simulink model "Performance_QP_Simulink"  (R2021a)
settings: Solver=ode45  StartTime=0.0  StopTime=20  FixedStep=Control_timestep  RelTol=1e-3  AbsTol=1e-6
undefined symbols (not defined in the file): Matlab_version, NXMotion, NXMotion_controltimestep, NXMotion_model, NXMotion_model_n, NXMotion_n, NXMotion_solution, NXMotion_solution_n, Plant_inputs_num, Plant_outputs_num
libraries: simulink x1
(part 2 of 3)

== matlab function Performance_QP_Simulink/MATLAB Function5 ==
  data: A input; B input; Theta0 input; XB input; P0 input; dh input; g output; q input; J input
function g = Performance_Gradient(A, B, Theta0, XB, P0, dh, q, J)
% 当前优化指标：
%   1) 世界坐标系 z 方向的 Directional Force Manipulability
%   2) 世界坐标系 x-y 平面的 Directional Velocity Transmission
%   3) 世界坐标系 rx-ry 平面的 Directional Rotational Stiffness


    %% -------------------------------------------------
    % 0. 固定输出尺寸与输入整理
    % --------------------------------------------------
    g = zeros(13,1);

    mu_const = 5;

    q      = reshape(q,      13, 1);
    J      = reshape(J,       6, 13);
    A      = reshape(A,       6, 3);
    B      = reshape(B,       6, 3);
    XB     = reshape(XB,      3, 1);
    P0     = reshape(P0,      3, 1);
    dh     = reshape(dh,      7, 4);
    Theta0 = reshape(Theta0,  7, 1);

    theta7_fixed = 0.0;

    q(13)   = theta7_fixed;
    J(:,13) = 0.0;

    %% -------------------------------------------------
    % 1. 调参量
    % --------------------------------------------------
    dt = 1.0e-3;

    % z 方向 Directional Force Manipulability 权重
    w_m = 1;

    % rx-ry 方向 Rotational Stiffness 权重
    w_s = 0;

    % x-y 方向 Velocity Transmission 权重
    w_v = 0;

    % 离散加速度层缩放：
    %   q_{k+1} ≈ q_k + qdot_k*dt + 0.5*qddot_k*dt^2
    mu = mu_const * 0.5 * dt * dt;

    %% -------------------------------------------------
    % 2. 构造性能指标矩阵
    % --------------------------------------------------
    [S_tau, Kq_inv, S_qdot] = build_metric_mats_perf();

    %% -------------------------------------------------
    % 3. 当前构型下的 Jacobian 单位转换
    % --------------------------------------------------
    Jv_now = convert_Jv_force_velocity_units(J);
    Jk_now = convert_J_stiffness_units(J);

    %% -------------------------------------------------
    % 4. 当前性能指标相关中间量
    % --------------------------------------------------
    ez = [
        0.0;
        0.0;
        1.0
    ];

    ez = ez / max(norm(ez), 1.0e-12);

    %% 4.1 z 方向 Directional Force Manipulability
    %
    % eta_m,z = 1 / sqrt(ez' * Jv*S_tau*Jv' * ez)
    % --------------------------------------------------
    Mf = Jv_now * S_tau * Jv_now.';
    Mf = 0.5 * (Mf + Mf.');

    alpha_m = ez.' * Mf * ez;
    alpha_m = max(real(alpha_m), 1.0e-12);

    %% 4.2 rx-ry Rotational Stiffness
    %
    % Kx = inv(J*Kq_inv*J')
    % eta_s,rxy = lambda_min(KR(1:2,1:2))
    % --------------------------------------------------
    Ms = Jk_now * Kq_inv * Jk_now.';
    Ms = 0.5 * (Ms + Ms.');

    scale_Ms = 0.0;
    for r = 1:6
        for c = 1:6
            scale_Ms = scale_Ms + Ms(r,c) * Ms(r,c);
        end
    end
    scale_Ms = sqrt(scale_Ms);

    reg_s = 1.0e-10 * max(scale_Ms, 1.0);

    Kx = (Ms + reg_s * eye(6)) \ eye(6);
    Kx = 0.5 * (Kx + Kx.');

    KR = Kx(4:6,4:6);
    KR = 0.5 * (KR + KR.');

    KRxy = KR(1:2,1:2);
    KRxy = 0.5 * (KRxy + KRxy.');

    [lambda_s, u_s_2] = min_eig_sym_2x2_with_vec(KRxy);
    lambda_s = max(real(lambda_s), 1.0e-12); %#ok<NASGU>

    % y_s = E' * u_s，其中 E 选取 Kx 的第 4、5 行列，即 rx, ry。
    y_s = zeros(6,1);
    y_s(4) = u_s_2(1);
    y_s(5) = u_s_2(2);

    % d eta_s = y_s' * dKx * y_s
    % dKx = -Kx * dMs * Kx
    z_s = Kx * y_s;

    %% 4.3 x-y Velocity Transmission
    %
    % eta_v,xy = sqrt(lambda_min(Jxy*S_qdot*Jxy'))
    % --------------------------------------------------
    Jxy_now = Jv_now(1:2,:);

    Mv = Jxy_now * S_qdot * Jxy_now.';
    Mv = 0.5 * (Mv + Mv.');

    [lambda_v, u_v] = min_eig_sym_2x2_with_vec(Mv);
    lambda_v = max(real(lambda_v), 1.0e-12);

    eta_v = sqrt(lambda_v);
    eta_v = max(real(eta_v), 1.0e-12);

    %% -------------------------------------------------
    % 5. 差分步长
    % --------------------------------------------------
    h = zeros(13,1);

    h(1:6)  = 1.0e-2;   % Stewart 电缸，单位 mm
    h(7:12) = 1.0e-3;   % 机械臂关节，单位 deg
    h(13)   = 0.0;      

    qdot0 = zeros(13,1);

    %% -------------------------------------------------
    % 6. 梯度计算
    % --------------------------------------------------
    grad_eta_m_formula = zeros(13,1);
    grad_eta_s_formula = zeros(13,1);
    grad_eta_v_formula = zeros(13,1);

    grad_eta_m_fd = zeros(13,1);
    grad_eta_s_fd = zeros(13,1);
    grad_eta_v_fd = zeros(13,1);

    for i = 1:12

        qp = q;
        qm = q;

        qp(i) = qp(i) + h(i);
        qm(i) = qm(i) - h(i);

        % 第 7 机械臂关节固定
        qp(13) = theta7_fixed;
        qm(13) = theta7_fixed;

        [Jp_ext, ~] = System_Kinematics(A, B, XB, P0, dh, Theta0, qp, qdot0);
        [Jm_ext, ~] = System_Kinematics(A, B, XB, P0, dh, Theta0, qm, qdot0);

        Jp_ext = reshape(Jp_ext, 6, 13);
        Jm_ext = reshape(Jm_ext, 6, 13);

        Jp_ext(:,13) = 0.0;
        Jm_ext(:,13) = 0.0;

        %% -------------------------------------------------
        % 6.1 直接差分 eta，用于验证解析公式
        % --------------------------------------------------
        eta_m_p = eta_dfm_z_from_J_perf(Jp_ext, S_tau);
        eta_m_m = eta_dfm_z_from_J_perf(Jm_ext, S_tau);

        eta_s_p = eta_stiffness_rxy_from_J_perf(Jp_ext, Kq_inv);
        eta_s_m = eta_stiffness_rxy_from_J_perf(Jm_ext, Kq_inv);

        eta_v_p = eta_velocity_xy_from_J_perf(Jp_ext, S_qdot);
        eta_v_m = eta_velocity_xy_from_J_perf(Jm_ext, S_qdot);

        grad_eta_m_fd(i) = (eta_m_p - eta_m_m) / (2.0 * h(i));
        grad_eta_s_fd(i) = (eta_s_p - eta_s_m) / (2.0 * h(i));
        grad_eta_v_fd(i) = (eta_v_p - eta_v_m) / (2.0 * h(i));

        %% -------------------------------------------------
        % 6.2 dJ/dq_i，用于解析公式
        % --------------------------------------------------
        Jv_p = convert_Jv_force_velocity_units(Jp_ext);
        Jv_m = convert_Jv_force_velocity_units(Jm_ext);

        dJv_dqi = (Jv_p - Jv_m) / (2.0 * h(i));

        Jk_p = convert_J_stiffness_units(Jp_ext);
        Jk_m = convert_J_stiffness_units(Jm_ext);

        dJk_dqi = (Jk_p - Jk_m) / (2.0 * h(i));

        %% -------------------------------------------------
        % 6.3 z 方向 Directional Force Manipulability 解析梯度
        % --------------------------------------------------
        term_m = ez.' * (dJv_dqi * S_tau * Jv_now.') * ez;
        grad_eta_m_formula(i) = - real(term_m) / (alpha_m^(1.5));

        %% -------------------------------------------------
        % 6.4 rx-ry Rotational Stiffness 解析梯度
        % --------------------------------------------------
        dMs_dqi = dJk_dqi * Kq_inv * Jk_now.' ...
                + Jk_now * Kq_inv * dJk_dqi.';

        dMs_dqi = 0.5 * (dMs_dqi + dMs_dqi.');

        dreg_s = 0.0;

        if scale_Ms > 1.0
            dscale_Ms = 0.0;

            for r = 1:6
                for c = 1:6
                    dscale_Ms = dscale_Ms + Ms(r,c) * dMs_dqi(r,c);
                end
            end

            dscale_Ms = dscale_Ms / max(scale_Ms, 1.0e-12);
            dreg_s = 1.0e-10 * dscale_Ms;
        end

        dA_s = dMs_dqi + dreg_s * eye(6);

        grad_eta_s_formula(i) = - real(z_s.' * dA_s * z_s);

        %% -------------------------------------------------
        % 6.5 x-y Velocity Transmission 解析梯度
        % --------------------------------------------------
        dJxy_dqi = dJv_dqi(1:2,:);

        dMv_dqi = dJxy_dqi * S_qdot * Jxy_now.' ...
                + Jxy_now * S_qdot * dJxy_dqi.';

        dMv_dqi = 0.5 * (dMv_dqi + dMv_dqi.');

        grad_eta_v_formula(i) = ...
            real(u_v.' * dMv_dqi * u_v) / (2.0 * eta_v);

    end

    grad_eta_m_formula(13) = 0.0;
    grad_eta_s_formula(13) = 0.0;
    grad_eta_v_formula(13) = 0.0;

    grad_eta_m_fd(13) = 0.0;
    grad_eta_s_fd(13) = 0.0;
    grad_eta_v_fd(13) = 0.0;

    %% -------------------------------------------------
    % 8. 误差检查
    % --------------------------------------------------
    err_eta_m = grad_eta_m_formula - grad_eta_m_fd;
    err_eta_s = grad_eta_s_formula - grad_eta_s_fd;
    err_eta_v = grad_eta_v_formula - grad_eta_v_fd;

    idx_check = 1:12;

    err_m_abs = norm(err_eta_m(idx_check));
    err_s_abs = norm(err_eta_s(idx_check));
    err_v_abs = norm(err_eta_v(idx_check));

    err_m_rel = err_m_abs / max(norm(grad_eta_m_fd(idx_check)), 1.0e-12);
    err_s_rel = err_s_abs / max(norm(grad_eta_s_fd(idx_check)), 1.0e-12);
    err_v_rel = err_v_abs / max(norm(grad_eta_v_fd(idx_check)), 1.0e-12);

    grad_check = [
        err_m_abs;
        err_m_rel;
        err_s_abs;
        err_s_rel;
        err_v_abs;
        err_v_rel
    ];

    %% -------------------------------------------------
    % 9. 输出 QP 线性性能项
    % --------------------------------------------------
    grad_eta_m = grad_eta_m_formula;
    grad_eta_s = grad_eta_s_formula;
    grad_eta_v = grad_eta_v_formula;

    g = mu * ( ...
          w_m * grad_eta_m ...
        + w_s * grad_eta_s ...
        + w_v * grad_eta_v );

    g_fd = mu * ( ...
          w_m * grad_eta_m_fd ...
        + w_s * grad_eta_s_fd ...
        + w_v * grad_eta_v_fd );

    g(13) = 0.0;
    g_fd(13) = 0.0;

end

%% ========================================================================
%                    Performance metric matrices
% ========================================================================

function [S_tau, Kq_inv, S_qdot] = build_metric_mats_perf()

    %% 1. 执行器力/力矩归一化矩阵 S_tau
    F_lim_cyl = 0.7 * [
        30;
        30;
        30;
        30;
        30;
        30
    ];  % N

    tau_lim_arm_Nm = 0.7 * [
        87;
        87;
        87;
        87;
        12;
        12;
        12
    ];  % Nm

    tau_lim_arm = tau_lim_arm_Nm * 1000.0;  % N*mm

    tau_lim = [
        F_lim_cyl;
        tau_lim_arm
    ];

    inv_tau = zeros(13,1);

    for i = 1:13
        inv_tau(i) = 1.0 / max(tau_lim(i), 1.0e-9);
    end

    inv_tau(13) = 0.0;

    S_tau = diag(inv_tau .* inv_tau);

    %% 2. 关节刚度矩阵 Kq 的逆矩阵 Kq_inv
    k_cyl = 1.0e4 * [
        1;
        1;
        1;
        1;
        1;
        1
    ];  % N/mm

    k_arm_Nm_per_rad = 1.0e3 * [
        1;
        1;
        1;
        1;
        1;
        1;
        1
    ];  % Nm/rad

    k_arm = k_arm_Nm_per_rad * 1000.0;  % N*mm/rad

    k_joint = [
        k_cyl;
        k_arm
    ];

    inv_kq = zeros(13,1);

    for i = 1:13
        inv_kq(i) = 1.0 / max(k_joint(i), 1.0e-9);
    end

    inv_kq(13) = 0.0;

    Kq_inv = diag(inv_kq);

    %% 3. 关节速度能力矩阵 S_qdot
    ldot_lim = 30.0;       % mm/s
    qdot_arm_lim = 0.50;   % rad/s

    qdot_lim = [
        ldot_lim * ones(6,1);
        qdot_arm_lim * ones(7,1)
    ];

    qdot_lim(13) = 0.0;

    S_qdot = diag(qdot_lim .* qdot_lim);

end

%% ========================================================================
%                    Jacobian unit conversion for force and velocity
% ========================================================================

function Jv = convert_Jv_force_velocity_units(J_ext)

    J_ext = reshape(J_ext, 6, 13);

    rad2deg = 180.0 / pi;

    Jv = J_ext(1:3,:);

    % Arm 列由 mm/deg 转为 mm/rad
    Jv(:,7:13) = Jv(:,7:13) * rad2deg;

    % 第 7 机械臂关节固定
    Jv(:,13) = 0.0;

end

%% ========================================================================
%                    Jacobian unit conversion for stiffness
% ========================================================================

function Jk = convert_J_stiffness_units(J_ext)

    J_ext = reshape(J_ext, 6, 13);

    deg2rad = pi / 180.0;
    rad2deg = 180.0 / pi;

    Jk = J_ext;

    % 输出角速度/角位移单位：deg -> rad
    Jk(4:6,:) = Jk(4:6,:) * deg2rad;

    % 机械臂输入关节单位：deg -> rad
    Jk(:,7:13) = Jk(:,7:13) * rad2deg;

    % 第 7 机械臂关节固定
    Jk(:,13) = 0.0;

end

%% ========================================================================
%                    Direct eta functions for finite-difference check
% ========================================================================

function eta = eta_dfm_z_from_J_perf(J_ext, S_tau)

    J_ext = reshape(J_ext, 6, 13);
    S_tau = reshape(S_tau, 13, 13);

    ez = [
        0.0;
        0.0;
        1.0
    ];

    ez = ez / max(norm(ez), 1.0e-12);

    Jv = convert_Jv_force_velocity_units(J_ext);

    alpha = ez.' * (Jv * S_tau * Jv.') * ez;
    alpha = max(real(alpha), 1.0e-12);

    eta = 1.0 / sqrt(alpha);
    eta = real(eta);
    eta = max(eta, 1.0e-12);

end

function eta = eta_stiffness_rxy_from_J_perf(J_ext, Kq_inv)

    J_ext  = reshape(J_ext,   6, 13);
    Kq_inv = reshape(Kq_inv, 13, 13);

    Jk = convert_J_stiffness_units(J_ext);

    Cx = Jk * Kq_inv * Jk.';
    Cx = 0.5 * (Cx + Cx.');

    scale_C = 0.0;
    for r = 1:6
        for c = 1:6
            scale_C = scale_C + Cx(r,c) * Cx(r,c);
        end
    end
    scale_C = sqrt(scale_C);

    reg = 1.0e-10 * max(scale_C, 1.0);

    Kx = (Cx + reg * eye(6)) \ eye(6);
    Kx = 0.5 * (Kx + Kx.');

    KR = Kx(4:6,4:6);
    KR = 0.5 * (KR + KR.');

    KRxy = KR(1:2,1:2);
    KRxy = 0.5 * (KRxy + KRxy.');

    eta = min_eig_sym_2x2(KRxy);

    eta = real(eta);
    eta = max(eta, 1.0e-12);

end

function eta = eta_velocity_xy_from_J_perf(J_ext, S_qdot)

    J_ext  = reshape(J_ext,   6, 13);
    S_qdot = reshape(S_qdot, 13, 13);

    Jv = convert_Jv_force_velocity_units(J_ext);

    Jxy = Jv(1:2,:);

    Mv = Jxy * S_qdot * Jxy.';
    Mv = 0.5 * (Mv + Mv.');

    lambda_min = min_eig_sym_2x2(Mv);
    lambda_min = max(real(lambda_min), 1.0e-12);

    eta = sqrt(lambda_min);
    eta = real(eta);
    eta = max(eta, 1.0e-12);

end

%% ========================================================================
%                    2x2 symmetric min eigenvalue
% ========================================================================

function lambda_min = min_eig_sym_2x2(M)

    M = reshape(M, 2, 2);
    M = 0.5 * (M + M.');

    a = M(1,1);
    b = M(1,2);
    c = M(2,2);

    tr_half = 0.5 * (a + c);

    disc_arg = 0.25 * (a - c) * (a - c) + b * b;
    disc_arg = max(disc_arg, 0.0);

    disc = sqrt(disc_arg);

    lambda_min = tr_half - disc;

end

%% ========================================================================
%                    2x2 symmetric min eigenvalue and eigenvector
% ========================================================================

function [lambda_min, u_min] = min_eig_sym_2x2_with_vec(M)

    M = reshape(M, 2, 2);
    M = 0.5 * (M + M.');

    a = M(1,1);
    b = M(1,2);
    c = M(2,2);

    tr_half = 0.5 * (a + c);

    disc_arg = 0.25 * (a - c) * (a - c) + b * b;

    if disc_arg < 0.0
        disc_arg = 0.0;
    end

    disc = sqrt(disc_arg);

    lambda_min = tr_half - disc;

    % 求解对应特征向量
    v1 = b;
    v2 = lambda_min - a;

    nrm = sqrt(v1*v1 + v2*v2);

    if nrm < 1.0e-12

        if a <= c
            u_min = [
                1.0;
                0.0
            ];
        else
            u_min = [
                0.0;
                1.0
            ];
        end

    else
        u_min = [
            v1 / nrm;
            v2 / nrm
        ];
    end

end

== matlab function Performance_QP_Simulink/MATLAB Function6 ==
  data: qdot_cmd_output output; t input; A input; B input; Theta0 input; qddot_cmd input; q input; qdot_in input
function qdot_cmd_output  = Command_Integrator( ...
     t, A, B, Theta0, qddot_cmd, q, qdot_in)


    %% -------------------------------------------------
    % 0. 固定输出尺寸与输入整理
    % --------------------------------------------------
    qdot_cmd_output = zeros(12,1);

    qddot_cmd = reshape(qddot_cmd, 13, 1);
    q          = reshape(q,          13, 1);
    qdot_in    = reshape(qdot_in,    13, 1);
    A          = reshape(A,           6, 3);
    B          = reshape(B,           6, 3);

    %% -------------------------------------------------
    % 0.1 启动保护
    % --------------------------------------------------
    t_start = 2.0e-3;   % s

    if t < t_start
        qdot_cmd_output(:) = 0.0;
        return;
    end

    %% -------------------------------------------------
    % 1. Theta0 处理
    % --------------------------------------------------
    Theta0_vec = Theta0(:);
    nTheta0 = numel(Theta0_vec);

    if nTheta0 >= 7
        theta7_fixed = Theta0_vec(7);
    else
        theta7_fixed = Theta0_vec(1);
    end

    %% -------------------------------------------------
    % 2. 内部 13 维 qdot
    % --------------------------------------------------
    qdot = qdot_in;

    %% -------------------------------------------------
    % 3. 控制周期
    % --------------------------------------------------
    dt = 1.0000e-03;     % s

    %% -------------------------------------------------
    % 4. 由 A、B 计算 Stewart 初始长度 L0
    % --------------------------------------------------
    dAB = A - B;
    L0 = zeros(6,1);

    for i = 1:6
        L0(i) = sqrt(dAB(i,1)*dAB(i,1) + ...
                     dAB(i,2)*dAB(i,2) + ...
                     dAB(i,3)*dAB(i,3));
    end

    q(13)         = theta7_fixed;
    qdot(13)      = 0.0;
    qddot_cmd(13) = 0.0;

    rad2deg = 180.0 / pi;

    q_min = zeros(13,1);
    q_max = zeros(13,1);

    stroke_half = 100.0;     % mm

    q_min(1:6) = L0 - stroke_half;
    q_max(1:6) = L0 + stroke_half;

    theta_min_rad = [
        -2.8973;
        -1.7628;
        -2.8973;
        -3.0718;
        -2.8973;
        -0.0175;
        -2.8973
    ];

    theta_max_rad = [
         2.8973;
         1.7628;
         2.8973;
        -0.0698;
         2.8973;
         3.7525;
         2.8973
    ];

    theta_min = theta_min_rad * rad2deg;
    theta_max = theta_max_rad * rad2deg;

    q_min(7:13) = theta_min;
    q_max(7:13) = theta_max;

    q_min(13) = theta7_fixed;
    q_max(13) = theta7_fixed;

    qdot_min = zeros(13,1);
    qdot_max = zeros(13,1);

    ldot_max = 30.0;                % mm/s
    thetadot_max = 0.50 * rad2deg;  % deg/s

    qdot_min(1:6)  = -ldot_max;
    qdot_max(1:6)  =  ldot_max;

    qdot_min(7:12) = -thetadot_max;
    qdot_max(7:12) =  thetadot_max;

    qdot_min(13) = 0.0;
    qdot_max(13) = 0.0;

    qddot_min = zeros(13,1);
    qddot_max = zeros(13,1);

    lddot_max = 200.0;               % mm/s^2
    thetaddot_max = 1.00 * rad2deg;  % deg/s^2

    qddot_min(1:6)  = -lddot_max;
    qddot_max(1:6)  =  lddot_max;

    qddot_min(7:12) = -thetaddot_max;
    qddot_max(7:12) =  thetaddot_max;

    qddot_min(13) = 0.0;
    qddot_max(13) = 0.0;


    qddot_safe = sat_vec13(qddot_cmd, qddot_min, qddot_max);


    qdot_des = qdot + qddot_safe * dt;
    

    qdot_des = sat_vec13(qdot_des, qdot_min, qdot_max);


    qdot_cmd = zeros(13,1);

    for i = 1:13

        lb_pos = (q_min(i) - q(i)) / dt;
        ub_pos = (q_max(i) - q(i)) / dt;

        lb = max(qdot_min(i), lb_pos);
        ub = min(qdot_max(i), ub_pos);

        if lb <= ub
            qdot_cmd(i) = sat_scalar(qdot_des(i), lb, ub);
        else
            if q(i) < q_min(i)
                qdot_cmd(i) = qdot_max(i);
            elseif q(i) > q_max(i)
                qdot_cmd(i) = qdot_min(i);
            else
                qdot_cmd(i) = 0.0;
            end
        end
    end


    qdot_cmd(13) = 0.0;

    qdot_cmd_output(1:12) = qdot_cmd(1:12);


end

%% ========================================================================
%                         helper: 13x1 vector saturation
% ========================================================================

function y = sat_vec13(x, lb, ub)
    y = zeros(13,1);

    for i = 1:13
        y(i) = sat_scalar(x(i), lb(i), ub(i));
    end
end

%% ========================================================================
%                         helper: scalar saturation
% ========================================================================

function y = sat_scalar(x, lb, ub)

    if ~isfinite(x)
        x = 0.0;
    end

    if ~isfinite(lb)
        lb = -realmax;
    end

    if ~isfinite(ub)
        ub = realmax;
    end

    y = x;

    if y < lb
        y = lb;
    end

    if y > ub
        y = ub;
    end
end

== matlab function Performance_QP_Simulink/MATLAB Function7 ==
  data: t input; Xddot_des input; A input; B input; Theta0 input; g input; q input; qdot_in input; J input; Jdot_qdot input; qddot_cmd output; eta_m_z output; eta_s_rxy output; eta_v_xy output
function [qddot_cmd, eta_m_z, eta_s_rxy, eta_v_xy] = QP_Builder_Solver( ...
     t, Xddot_des, A, B, Theta0, g, q, qdot_in, J, Jdot_qdot)

    %% -------------------------------------------------
    % 0. 固定输出尺寸与输入整理
    % --------------------------------------------------
    qddot_cmd = zeros(13,1);

    J          = reshape(J,          6, 13);
    Jdot_qdot = reshape(Jdot_qdot,   6, 1);
    Xddot_des = reshape(Xddot_des,   6, 1);
    g          = reshape(g,         13, 1);
    q          = reshape(q,         13, 1);
    qdot_in    = reshape(qdot_in,   13, 1);
    A          = reshape(A,          6, 3);
    B          = reshape(B,          6, 3);

    eta_m_z   = 0.0;
    eta_s_rxy = 0.0;
    eta_v_xy  = 0.0;

    %% -------------------------------------------------
    % 0.1 启动保护
    % --------------------------------------------------
    t_start = 2.0e-3;   % s

    if t < t_start
        qddot_cmd(:) = 0.0;
        return;
    end

    %% -------------------------------------------------
    % 0.2 NaN / Inf 保护
    % --------------------------------------------------
    if has_bad_mat_6x13(J) || has_bad_vec6(Jdot_qdot) || has_bad_vec6(Xddot_des)
        qddot_cmd(:) = 0.0;
        return;
    end

    % 兼容 Theta0 为 7x1 或 1x1 的情况
    Theta0_vec = Theta0(:);
    if numel(Theta0_vec) >= 7
        theta7_fixed = Theta0_vec(7);
    else
        theta7_fixed = Theta0_vec(1);
    end


    qdot = qdot_in;

    q(13)     = theta7_fixed;
    qdot(13)  = 0.0;
    J(:,13)   = 0.0;
    g(13)     = 0.0;


    
    %% -------------------------------------------------
    % 1. 控制周期
    % --------------------------------------------------
    dt = 1.0000e-03;     % s

    %% -------------------------------------------------
    % 2. 单位转换矩阵
    % --------------------------------------------------
    mm_to_m = 1.0e-3;
    m_to_mm = 1.0e3;

    deg2rad = pi / 180.0;
    rad2deg = 180.0 / pi;

    Dq = diag([
        mm_to_m;
        mm_to_m;
        mm_to_m;
        mm_to_m;
        mm_to_m;
        mm_to_m;
        deg2rad;
        deg2rad;
        deg2rad;
        deg2rad;
        deg2rad;
        deg2rad;
        deg2rad
    ]);

    Dq_inv = diag([
        m_to_mm;
        m_to_mm;
        m_to_mm;
        m_to_mm;
        m_to_mm;
        m_to_mm;
        rad2deg;
        rad2deg;
        rad2deg;
        rad2deg;
        rad2deg;
        rad2deg;
        rad2deg
    ]);

    Dx = diag([
        mm_to_m;
        mm_to_m;
        mm_to_m;
        deg2rad;
        deg2rad;
        deg2rad
    ]);

    %% -------------------------------------------------
    % 3. 转换到内部 m/rad 单位
    % --------------------------------------------------
    J_phy = Dx * J * Dq_inv;

    Jdot_qdot_phy = Dx * Jdot_qdot;
    Xddot_des_phy = Dx * Xddot_des;

    g_phy = Dq_inv.' * g;

    J_phy(:,13) = 0.0;
    g_phy(13) = 0.0;

    %% -------------------------------------------------
    % 3.1 当前性能指标计算
    % --------------------------------------------------
    [S_tau_metric, Kq_inv_metric, S_qdot_metric] = build_metric_mats_qp();

    eta_m_z   = eta_dfm_z_from_J_qp(J, S_tau_metric);
    eta_s_rxy = eta_stiffness_rxy_from_J_qp(J, Kq_inv_metric);
    eta_v_xy  = eta_velocity_xy_from_J_qp(J, S_qdot_metric);

    if ~isfinite(eta_m_z)
        eta_m_z = 0.0;
    end

    if ~isfinite(eta_s_rxy)
        eta_s_rxy = 0.0;
    end

    if ~isfinite(eta_v_xy)
        eta_v_xy = 0.0;
    end

    %% -------------------------------------------------
    % 3.2 固定短时间窗口启用 g，并限制 g 的关节分配
    % --------------------------------------------------

    g_window_start = 0.020;    % s
    g_window_end   = 5;    % s
    g_ramp_time    = 0.100;    % s

    gamma_g = 0.0;

    window_len = g_window_end - g_window_start;

    if window_len <= 1.0e-9
        gamma_g = 0.0;
    else
        if g_ramp_time > 0.5 * window_len
            g_ramp = 0.5 * window_len;
        else
            g_ramp = g_ramp_time;
        end

        if g_ramp <= 1.0e-9
            if t >= g_window_start && t <= g_window_end
                gamma_g = 1.0;
            else
                gamma_g = 0.0;
            end
        else
            if t < g_window_start
                gamma_g = 0.0;

            elseif t < g_window_start + g_ramp
                gamma_g = (t - g_window_start) / g_ramp;

            elseif t <= g_window_end - g_ramp
                gamma_g = 1.0;

            elseif t < g_window_end
                gamma_g = (g_window_end - t) / g_ramp;

            else
                gamma_g = 0.0;
            end
        end
    end

    if gamma_g < 0.0
        gamma_g = 0.0;
    end

    if gamma_g > 1.0
        gamma_g = 1.0;
    end

    % ---------- g 的关节分量缩放 ----------

    g_scale = zeros(13,1);

    g_scale(1:6) = 0.1;

    g_scale(7:12) = 0.1;

    g_phy = gamma_g * (g_scale .* g_phy);

    g_phy(13) = 0.0;

    %% -------------------------------------------------
    % 4. QP 权重矩阵
    % --------------------------------------------------
    Wx = diag([
        1.0;
        1.0;
        3.0;
        0.2;
        0.2;
        0.2
    ]);

    Wq_diag = zeros(13,1);
  
    Wq_diag(1:6)   = 1.0e-3;   
    Wq_diag(7:12)  = 1.0e-4;   
    Wq_diag(13)    = 1.0;      
    Wq = diag(Wq_diag);

    %% -------------------------------------------------
    % 5. 构造 QP 标准形式
    % --------------------------------------------------
    b_phy = Xddot_des_phy - Jdot_qdot_phy;

    H = 2.0 * (J_phy.' * Wx * J_phy + Wq);
    f = -2.0 * (J_phy.' * Wx * b_phy) - g_phy;

    H = 0.5 * (H + H.') + 1.0e-9 * eye(13);

    if has_bad_mat_13x13(H) || has_bad_vec13(f)
        qddot_cmd(:) = 0.0;
        return;
    end

    %% -------------------------------------------------
    % 6. 关节位置、速度、加速度限制
    % --------------------------------------------------
    dAB = A - B;
    L0 = sqrt(sum(dAB.^2, 2));       % 6x1, mm

    q_min = zeros(13,1);
    q_max = zeros(13,1);

    stroke = 800.0;     % mm

    q_min(1:6) = L0 - stroke;
    q_max(1:6) = L0 + stroke;

    theta_min_rad = [
        -2.8973;
        -1.7628;
        -2.8973;
        -3.0718;
        -2.8973;
        -0.0175;
        -2.8973
    ];

    theta_max_rad = [
         2.8973;
         1.7628;
         2.8973;
        -0.0698;
         2.8973;
         3.7525;
         2.8973
    ];

    theta_min = theta_min_rad * rad2deg;
    theta_max = theta_max_rad * rad2deg;

    q_min(7:13) = theta_min;
    q_max(7:13) = theta_max;

    q_min(13) = theta7_fixed;
    q_max(13) = theta7_fixed;

    qdot_min = zeros(13,1);
    qdot_max = zeros(13,1);

    ldot_max = 30.0;                  % mm/s
    thetadot_max = 0.50 * rad2deg;    % deg/s

    qdot_min(1:6)  = -ldot_max;
    qdot_max(1:6)  =  ldot_max;

    qdot_min(7:12) = -thetadot_max;
    qdot_max(7:12) =  thetadot_max;

    qdot_min(13) = 0.0;
    qdot_max(13) = 0.0;

    qddot_min = zeros(13,1);
    qddot_max = zeros(13,1);

    lddot_max = 200.0;                % mm/s^2
    thetaddot_max = 1.00 * rad2deg;   % deg/s^2

    qddot_min(1:6)  = -lddot_max;
    qddot_max(1:6)  =  lddot_max;

    qddot_min(7:12) = -thetaddot_max;
    qddot_max(7:12) =  thetaddot_max;

    qddot_min(13) = 0.0;
    qddot_max(13) = 0.0;

    %% -------------------------------------------------
    % 7. 转换为 qddot 上下界
    % --------------------------------------------------
    lb_ext = zeros(13,1);
    ub_ext = zeros(13,1);

    for i = 1:13
        lb_acc = qddot_min(i);
        ub_acc = qddot_max(i);

        lb_vel = (qdot_min(i) - qdot(i)) / dt;
        ub_vel = (qdot_max(i) - qdot(i)) / dt;

        lb_pos = 2.0 * (q_min(i) - q(i) - qdot(i)*dt) / (dt*dt);
        ub_pos = 2.0 * (q_max(i) - q(i) - qdot(i)*dt) / (dt*dt);

        lb_ext(i) = max(lb_acc, max(lb_vel, lb_pos));
        ub_ext(i) = min(ub_acc, min(ub_vel, ub_pos));
    end

    lb_ext(13) = 0.0;
    ub_ext(13) = 0.0;

    % 若当前状态已经越界导致 lb > ub，使用制动加速度保底
    for i = 1:13
        if lb_ext(i) > ub_ext(i)
            brake = -qdot(i) / dt;

            if brake < qddot_min(i)
                brake = qddot_min(i);
            end

            if brake > qddot_max(i)
                brake = qddot_max(i);
            end

            lb_ext(i) = brake;
            ub_ext(i) = brake;
        end
    end

    lb_ext(13) = 0.0;
    ub_ext(13) = 0.0;

    %% -------------------------------------------------
    % 8. 转换为内部单位
    % --------------------------------------------------
    lb_phy = Dq * lb_ext;
    ub_phy = Dq * ub_ext;

    %% -------------------------------------------------
    % 9. 求解带上下界约束的 QP
    % --------------------------------------------------
    qddot_phy = box_qp_projected_gradient_13(H, f, lb_phy, ub_phy);

    if has_bad_vec13(qddot_phy)
        qddot_cmd(:) = 0.0;
        return;
    end

    qddot_cmd = Dq_inv * qddot_phy;

    qddot_cmd = project_box_13(qddot_cmd, lb_ext, ub_ext);

    qddot_cmd(13) = 0.0;

end



%% ========================================================================
%                    Bound-constrained QP solver
% ========================================================================

function x = box_qp_projected_gradient_13(H, f, lb, ub)

    x = zeros(13,1);

    x0 = -(H \ f);

    if has_bad_vec13(x0)
        x0 = zeros(13,1);
    end

    x = project_box_13(x0, lb, ub);

    L = 0.0;
    for i = 1:13
        for j = 1:13
            L = L + H(i,j) * H(i,j);
        end
    end

    L = sqrt(L);

    if L < 1.0e-12
        L = 1.0;
    end

    alpha = 1.0 / L;

    maxIter = 100;
    tol = 1.0e-8;

    for k = 1:maxIter
        grad = H * x + f;

        x_new = project_box_13(x - alpha * grad, lb, ub);

        dx = x_new - x;

        if sqrt(sum(dx.^2)) <= tol * (1.0 + sqrt(sum(x.^2)))
            x = x_new;
            break;
        end

        x = x_new;
    end

end

%% ========================================================================
%                    Projection onto box constraints
% ========================================================================

function y = project_box_13(x, lb, ub)

    y = zeros(13,1);

    for i = 1:13
        yi = x(i);

        if yi < lb(i)
            yi = lb(i);
        end

        if yi > ub(i)
            yi = ub(i);
        end

        y(i) = yi;
    end

end

%% ========================================================================
%                    Performance metric matrices
% ========================================================================

function [S_tau, Kq_inv, S_qdot] = build_metric_mats_qp()

    %% -------------------------------------------------
    % 1. 执行器力/力矩归一化矩阵 S_tau
    % --------------------------------------------------
    F_lim_cyl = 0.7 * [
        30;
        30;
        30;
        30;
        30;
        30
    ];  % N

    tau_lim_arm_Nm = 0.7 * [
        87;
        87;
        87;
        87;
        12;
        12;
        12
    ];  % Nm

    tau_lim_arm = tau_lim_arm_Nm * 1000.0;  % N*mm

    tau_lim = [
        F_lim_cyl;
        tau_lim_arm
    ];

    inv_tau = zeros(13,1);

    for i = 1:13
        inv_tau(i) = 1.0 / max(tau_lim(i), 1.0e-9);
    end

    % 第 7 机械臂关节固定
    inv_tau(13) = 0.0;

    S_tau = diag(inv_tau .* inv_tau);

    %% -------------------------------------------------
    % 2. 关节刚度矩阵 Kq 的逆矩阵 Kq_inv
    % --------------------------------------------------
    k_cyl = 1.0e4 * [
        1;
        1;
        1;
        1;
        1;
        1
    ];  % N/mm

    k_arm_Nm_per_rad = 1.0e3 * [
        1;
        1;
        1;
        1;
        1;
        1;
        1
    ];  % Nm/rad

    k_arm = k_arm_Nm_per_rad * 1000.0;  % N*mm/rad

    k_joint = [
        k_cyl;
        k_arm
    ];

    inv_kq = zeros(13,1);

    for i = 1:13
        inv_kq(i) = 1.0 / max(k_joint(i), 1.0e-9);
    end

    % 第 7 机械臂关节固定
    inv_kq(13) = 0.0;

    Kq_inv = diag(inv_kq);

    %% -------------------------------------------------
    % 3. 关节速度能力矩阵 S_qdot
    % --------------------------------------------------
    ldot_lim = 30.0;       % mm/s
    qdot_arm_lim = 0.50;   % rad/s

    qdot_lim = [
        ldot_lim * ones(6,1);
        qdot_arm_lim * ones(7,1)
    ];

    % 第 7 机械臂关节固定
    qdot_lim(13) = 0.0;

    S_qdot = diag(qdot_lim .* qdot_lim);

end

%% ========================================================================
%                    z-direction force manipulability
% ========================================================================

function eta = eta_dfm_z_from_J_qp(J_ext, S_tau)

    J_ext = reshape(J_ext, 6, 13);
    S_tau = reshape(S_tau, 13, 13);

    rad2deg = 180.0 / pi;

    ez = [
        0.0;
        0.0;
        1.0
    ];

    ez = ez / max(norm(ez), 1.0e-12);

    Jv = J_ext(1:3,:);

    % Arm 列由 mm/deg 转为 mm/rad
    Jv(:,7:13) = Jv(:,7:13) * rad2deg;

    % 第 7 机械臂关节固定
    Jv(:,13) = 0.0;

    alpha = ez.' * (Jv * S_tau * Jv.') * ez;
    alpha = max(alpha, 1.0e-12);

    eta = 1.0 / sqrt(alpha);
    eta = real(eta);
    eta = max(eta, 1.0e-12);

end

%% ========================================================================
%                    rx-ry rotational stiffness
% ========================================================================

function eta = eta_stiffness_rxy_from_J_qp(J_ext, Kq_inv)

    J_ext  = reshape(J_ext,   6, 13);
    Kq_inv = reshape(Kq_inv, 13, 13);

    deg2rad = pi / 180.0;
    rad2deg = 180.0 / pi;

    Jk = J_ext;

    % 输出角速度/角位移单位：deg -> rad
    Jk(4:6,:) = Jk(4:6,:) * deg2rad;

    % 机械臂输入关节单位：deg -> rad
    Jk(:,7:13) = Jk(:,7:13) * rad2deg;

    % 第 7 机械臂关节固定
    Jk(:,13) = 0.0;

    Cx = Jk * Kq_inv * Jk.';
    Cx = 0.5 * (Cx + Cx.');

    scale_C = 0.0;
    for r = 1:6
        for c = 1:6
            scale_C = scale_C + Cx(r,c) * Cx(r,c);
        end
    end
    scale_C = sqrt(scale_C);

    reg = 1.0e-10 * max(scale_C, 1.0);

    Kx = (Cx + reg * eye(6)) \ eye(6);
    Kx = 0.5 * (Kx + Kx.');

    KR = Kx(4:6,4:6);
    KR = 0.5 * (KR + KR.');

    KRxy = KR(1:2,1:2);
    KRxy = 0.5 * (KRxy + KRxy.');

    eta = min_eig_sym_2x2_qp(KRxy);

    eta = real(eta);
    eta = max(eta, 1.0e-12);

end

%% ========================================================================
%                    x-y velocity transmission
% ========================================================================

function eta = eta_velocity_xy_from_J_qp(J_ext, S_qdot)

    J_ext  = reshape(J_ext,   6, 13);
    S_qdot = reshape(S_qdot, 13, 13);

    rad2deg = 180.0 / pi;

    Jv = J_ext(1:3,:);

    % Arm 列由 mm/deg 转为 mm/rad
    Jv(:,7:13) = Jv(:,7:13) * rad2deg;

    % 第 7 机械臂关节固定
    Jv(:,13) = 0.0;

    Jxy = Jv(1:2,:);

    Mv = Jxy * S_qdot * Jxy.';
    Mv = 0.5 * (Mv + Mv.');

    lambda_min = min_eig_sym_2x2_qp(Mv);
    lambda_min = max(real(lambda_min), 1.0e-12);

    eta = sqrt(lambda_min);
    eta = real(eta);
    eta = max(eta, 1.0e-12);

end

%% ========================================================================
%                    2x2 symmetric min eigenvalue
% ========================================================================

function lambda_min = min_eig_sym_2x2_qp(M)

    M = reshape(M, 2, 2);
    M = 0.5 * (M + M.');

    a = M(1,1);
    b = M(1,2);
    c = M(2,2);

    tr_half = 0.5 * (a + c);
    disc = sqrt(0.25 * (a - c) * (a - c) + b * b);

    lambda_min = tr_half - disc;

end

%% ========================================================================
%                    finite checks
% ========================================================================

function bad = has_bad_vec6(x)
    bad = false;
    for i = 1:6
        if ~isfinite(x(i))
            bad = true;
            return;
        end
    end
end

function bad = has_bad_vec13(x)
    bad = false;
    for i = 1:13
        if ~isfinite(x(i))
            bad = true;
            return;
        end
    end
end

function bad = has_bad_mat_6x13(A)
    bad = false;
    for i = 1:6
        for j = 1:13
            if ~isfinite(A(i,j))
                bad = true;
                return;
            end
        end
    end
end

function bad = has_bad_mat_13x13(A)
bad = false;
for i = 1:13
    for j = 1:13
        if ~isfinite(A(i,j))
            bad = true;
            return;
        end
    end
end
end
